simulink model "teset"  (R2016a)
settings: Solver=VariableStepAuto  StartTime=0.0  StopTime=10.0  RelTol=1e-3
settings Model: Creator=shohei  LastModifiedBy=shohei

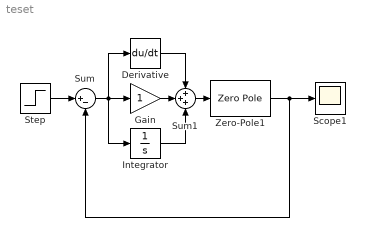
== system teset ==
  Derivative : Derivative  CoefficientInTFapproximation=Inf
  Gain : Gain
  Integrator : Integrator
  Scope1 : Scope
  Step : Step  SampleTime=0
  Sum : Sum  Inputs=|+-
  Sum1 : Sum  Inputs=+++
  Zero-Pole1 : ZeroPole  Poles=[0 -1]  Gain=[2]
  wires:
  Zero-Pole1/1 -> Sum/2, Scope1/1
  Step/1 -> Sum/1
  Sum1/1 -> Zero-Pole1/1
  Gain/1 -> Sum1/2
  Sum/1 -> Integrator/1, Derivative/1, Gain/1
  Integrator/1 -> Sum1/3
  Derivative/1 -> Sum1/1
